simulink model "NL_After_OHC_Function_fil"  (R2019b)
settings: Solver=VariableStepAuto  StartTime=0.0  StopTime=testtime  RelTol=1e-3
InitFcn:
  | NL_After_OHC_Test_Parameters
StopFcn:
  | Verify_NL_After_OHC_Function_fil
undefined symbols (not defined in the file or in its folder): Fs, minR, ohcasym, taumax, taumin
libraries: dspsrcs4 x2, simulink x1, hdlmdlgenlib x1, fillib x1
settings Model: Creator=mblun  LastModifiedBy=t96f346
settings OptimizationCC: BlockReduction=off  ConditionallyExecuteInputs=off  DefaultParameterBehavior=Inlined
settings DebuggingCC: AlgebraicLoopMsg=error  InheritedTsInSrcMsg=none
settings HardwareCC: ProdBitPerPointer=32  ProdBitPerSizeT=32  ProdBitPerPtrDiffT=32  ProdLargestAtomicFloat=None  ProdIntDivRoundTo=Undefined  ProdEndianess=Unspecified  ProdWordSize=32  ProdHWDeviceType=ASIC/FPGA->ASIC/FPGA  TargetBitPerPointer=64  TargetBitPerSizeT=64  TargetBitPerPtrDiffT=64  TargetLongLongMode=on  TargetIntDivRoundTo=Zero  TargetEndianess=LittleEndian  TargetWordSize=64  TargetHWDeviceType=Custom Processor->MATLAB Host Computer  ProdEqTarget=off
settings SFSimCC: CustomCodeUndefinedFunction=UseInterfaceOnly

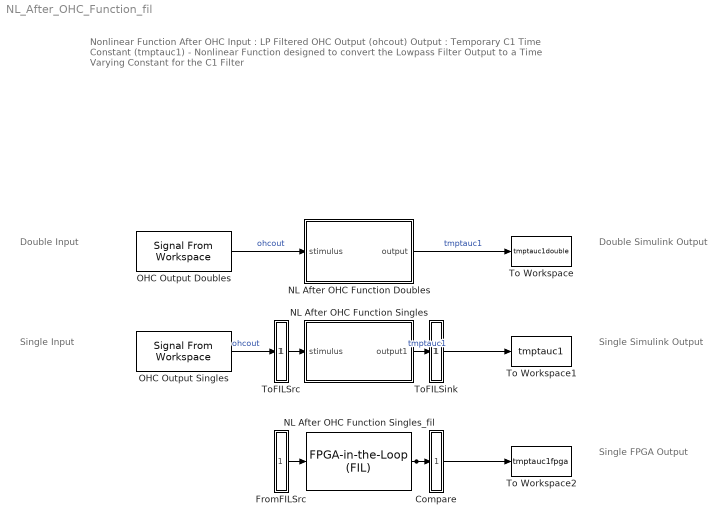
== system NL_After_OHC_Function_fil ==
  note: Nonlinear Function After OHC
      |
      | Input : LP Filtered OHC Output (ohcout)
      |
      | Output : Temporary C1 Time Constant (tmptauc1)
      |
      | - Nonlinear Function designed to convert the Lowpass Filter Output to a Time Varying Constant for the C1 Filter
  note: Single Input
  note: Double Input
  note: Single Simulink Output
  note: Double Simulink Output
  note: Single FPGA Output
  Compare : Subsystem
      mask Display: disp('')
  FromFILSrc : Subsystem
      mask Display: disp('')
  NL After OHC Function Doubles : Subsystem
  NL After OHC Function Singles : Subsystem
  NL After OHC Function Singles_fil : fillib/FPGA-in-the-Loop (FIL)  ForceInterfaceUpdate=0.91338
      settings: SourceProductName=HDL Coder  SourceProductBaseCode=HD
  OHC Output Doubles : dspsrcs4/Signal From Workspace  X=RxSignalDouble  Ts=1/Fs  nsamps=1  OutputAfterFinalValue=Setting to zero  ignoreOrWarnInputAndFrameLengths=off  OutputFrames=off
  OHC Output Singles : dspsrcs4/Signal From Workspace  X=RxSignal  Ts=1/Fs  nsamps=1  OutputAfterFinalValue=Setting to zero  ignoreOrWarnInputAndFrameLengths=off  OutputFrames=off
  To Workspace : ToWorkspace  VariableName=tmptauc1double  SampleTime=-1
      settings: Save2DSignal=2-D array (concatenate along first dimension)
  To Workspace1 : ToWorkspace  VariableName=tmptauc1  SampleTime=-1
      settings: Save2DSignal=2-D array (concatenate along first dimension)
  To Workspace2 : ToWorkspace  VariableName=tmptauc1fpga  SampleTime=-1
      settings: Save2DSignal=2-D array (concatenate along first dimension)
  ToFILSink : Subsystem
      mask Display: disp('')
  ToFILSrc : Subsystem
      mask Display: disp('')
  wires:
  OHC Output Doubles/1 -> NL After OHC Function Doubles/1(stimulus)  "ohcout"
  NL After OHC Function Doubles/1(output) -> To Workspace/1  "tmptauc1"
  ToFILSrc/1(out1) -> NL After OHC Function Singles/1(stimulus)
  NL After OHC Function Singles/1(output1) -> ToFILSink/1(in1)  "tmptauc1"
  OHC Output Singles/1 -> ToFILSrc/1(in1)  "ohcout"
  ToFILSink/1(out1) -> To Workspace1/1
  FromFILSrc/1(out1) -> NL After OHC Function Singles_fil/1
  NL After OHC Function Singles_fil/1 -> To Workspace2/1, Compare/1(in1)

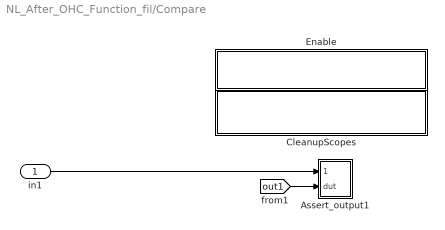
== system NL_After_OHC_Function_fil/Compare ==
  in1 : Inport
  Assert_output1 : Subsystem  mask{ToleranceValue=1e-07}
  CleanupScopes : Subsystem
      settings: OpenFcn=|
      | blkName = gcb; %self block
      | idx = regexp(blkName, '/CleanupScopes$', 'once');
      | blkParent = blkName(1:idx-1);
      | blks=find_system(blkParent, 'LookUnderMasks', 'all','blocktype', 'Scope');
      | for itr = 1:length(blks)
      | 	 hScopeCfg = get_param(blks{itr},'ScopeConfiguration');
      | 	 hScopeCfg.Visible = ~ hScopeCfg.Visible;
      | end
      | drawnow;
      mask Display: fprintf(message('hdlcoder:cosim:vnl_dblclick').getString());
  Enable : Subsystem
      settings: OpenFcn=|
      | blkName = gcb;
      | idx = regexp(blkName, '/Enable$', 'once');
      | blkParent = blkName(1:idx-1);
      | blks=find_system(blkParent, 'LookUnderMasks', 'all','blocktype', 'Assertion');
      | e = get_param(blks{1}, 'Enabled');
      | if strcmp(e, 'on'), f= 'off';, else, f = 'on';, end
      | for ii=1:length(blks), set_param(blks{ii}, 'Enabled', f);, end
      | set_param(gcb, 'MaskDisplay',['fprintf(message(''hdlcoder:cosim:vnl_dblclick_assertions'',','''',upper(e),'''',').getString())']);
      mask Display: fprintf(message('hdlcoder:cosim:vnl_dblclick_assertions','OFF').getString());
  wires:
  in1/1 -> Assert_output1/1(cosim)
  [out1] -> Assert_output1/2(dut)

== system NL_After_OHC_Function_fil/FromFILSrc ==
  dtc1 : DataTypeConversion  OutDataTypeStr=single  SaturateOnIntegerOverflow=on  RndMeth=Zero
  out1 : Outport
  wires:
  [in1] -> dtc1/1
  dtc1/1 -> out1/1

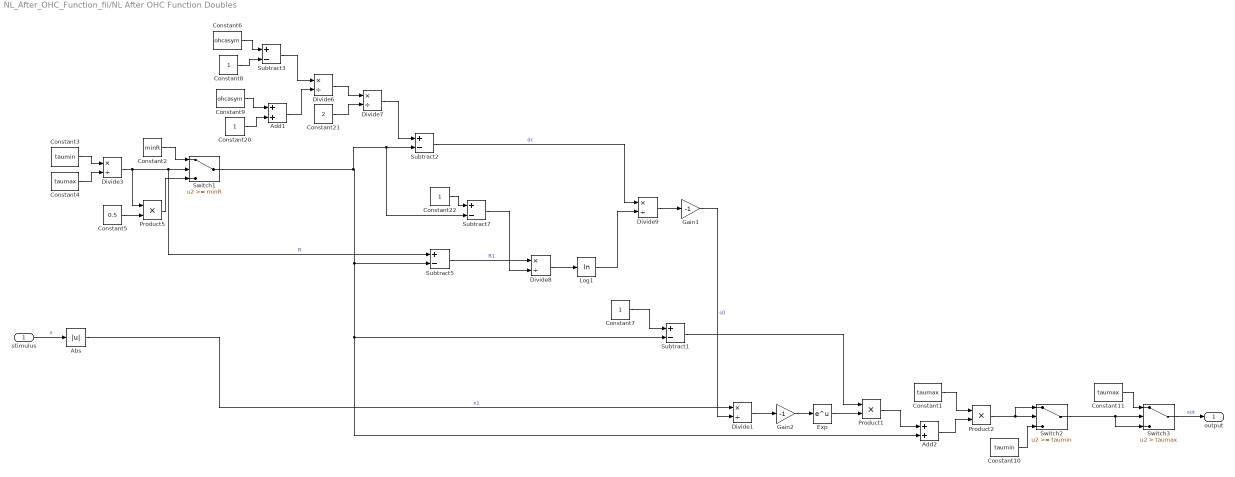
== system NL_After_OHC_Function_fil/NL After OHC Function Doubles ==
  stimulus : Inport
  Abs : Abs
  Add1 : Sum
  Add2 : Sum
  Constant1 : Constant  Value=taumax  SampleTime=-1
  Constant10 : Constant  Value=taumin  SampleTime=-1
  Constant11 : Constant  Value=taumax  SampleTime=-1
  Constant2 : Constant  Value=minR  SampleTime=-1
  Constant{7..8,20,22} (4 alike) : Constant  SampleTime=-1
  Constant21 : Constant  Value=2  SampleTime=-1
  Constant3 : Constant  Value=taumin  SampleTime=-1
  Constant4 : Constant  Value=taumax  SampleTime=-1
  Constant5 : Constant  Value=0.5  SampleTime=-1
  Constant6 : Constant  Value=ohcasym  SampleTime=-1
  Constant9 : Constant  Value=ohcasym  SampleTime=-1
  Divide{1,3,6..9} (6 alike) : Product  Inputs=*/  SaturateOnIntegerOverflow=on  RndMeth=Zero
  Exp : Math  SaturateOnIntegerOverflow=on
  Gain1 : Gain  Gain=-1
  Gain2 : Gain  Gain=-1
  Log1 : Math  Operator=log  SaturateOnIntegerOverflow=on
  Product1 : Product
  Product2 : Product
  Product5 : Product
  Subtract{1..3,5,7} (5 alike) : Sum  Inputs=+-
  Switch1 : Switch  Threshold=minR
  Switch2 : Switch  Threshold=taumin
  Switch3 : Switch  Criteria=u2 > Threshold  Threshold=taumax
  output : Outport  VectorParamsAs1DForOutWhenUnconnected=off
  wires:
  Constant3/1 -> Divide3/1
  Constant4/1 -> Divide3/2
  Divide3/1 -> Subtract5/1, Switch1/2, Product5/1  "R"
  Constant2/1 -> Switch1/1
  Constant5/1 -> Product5/2
  Product5/1 -> Switch1/3
  Switch1/1 -> Subtract7/2, Subtract2/2, Add2/2, Subtract1/2, Subtract5/2
  Constant8/1 -> Subtract3/2
  Constant6/1 -> Subtract3/1
  Constant20/1 -> Add1/2
  Constant9/1 -> Add1/1
  Subtract3/1 -> Divide6/1
  Add1/1 -> Divide6/2
  Divide6/1 -> Divide7/1
  Constant21/1 -> Divide7/2
  Divide7/1 -> Subtract2/1
  Subtract2/1 -> Divide9/1  "dc"
  Subtract5/1 -> Divide8/1  "R1"
  Constant22/1 -> Subtract7/1
  Subtract7/1 -> Divide8/2
  Divide8/1 -> Log1/1
  Log1/1 -> Divide9/2
  Divide9/1 -> Gain1/1
  Gain1/1 -> Divide1/2  "s0"
  stimulus/1 -> Abs/1  "x"
  Abs/1 -> Divide1/1  "x1"
  Constant7/1 -> Subtract1/1
  Divide1/1 -> Gain2/1
  Gain2/1 -> Exp/1
  Subtract1/1 -> Product1/1
  Exp/1 -> Product1/2
  Product1/1 -> Add2/1
  Constant1/1 -> Product2/1
  Add2/1 -> Product2/2
  Product2/1 -> Switch2/1, Switch2/2
  Constant10/1 -> Switch2/3
  Switch2/1 -> Switch3/3, Switch3/2
  Constant11/1 -> Switch3/1
  Switch3/1 -> output/1  "out"

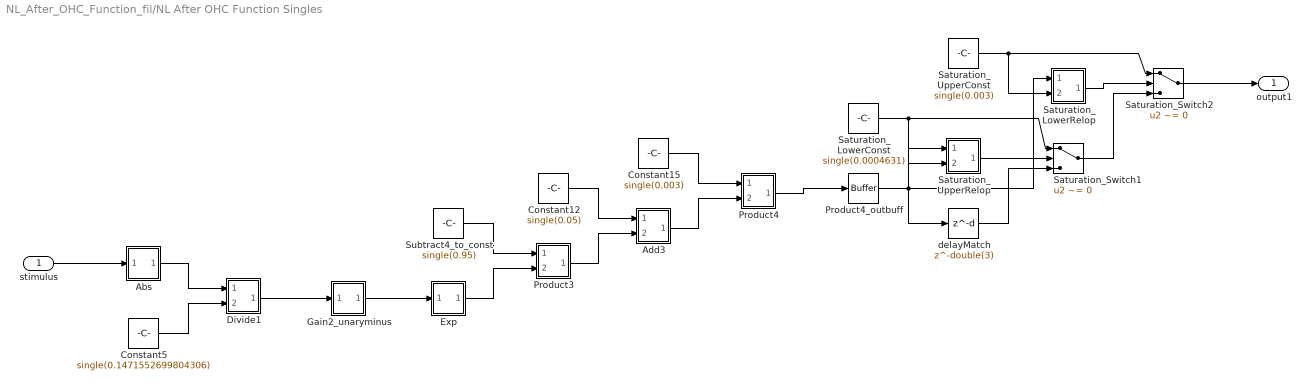
== system NL_After_OHC_Function_fil/NL After OHC Function Singles ==
  stimulus : Inport  OutDataTypeStr=single  PortDimensions=1  SampleTime=2.08333333333333e-05
  Abs : Subsystem
      mask Display: disp('NFP\nabs');
  Add3 : Subsystem
      mask Display: disp('NFP\nadd');
  Constant12 : Constant  Value=single(0.05)  OutDataTypeStr=single  SampleTime=-1
  Constant15 : Constant  Value=single(0.003)  OutDataTypeStr=single  SampleTime=-1
  Constant5 : Constant  Value=single(0.1471552699804306)  OutDataTypeStr=single  SampleTime=-1
  Divide1 : Subsystem
      mask Display: disp('NFP\nmul');
  Exp : Subsystem
      mask Display: disp('NFP\nmath');
  Gain2_unaryminus : Subsystem
      mask Display: disp('NFP\numinus');
  Product3 : Subsystem
      mask Display: disp('NFP\nmul');
  Product4 : Subsystem
      mask Display: disp('NFP\nmul');
  Product4_outbuff : hdlmdlgenlib/Buffer
      settings: SourceProductName=Simulink  SourceProductBaseCode=SL
  Saturation_LowerConst : Constant  Value=single(0.0004631)  OutDataTypeStr=single  SampleTime=-1
  Saturation_LowerRelop : Subsystem
      mask Display: disp('NFP\nrelop');
  Saturation_Switch1 : Switch  Criteria=u2 ~= 0  Threshold=double(0)  OutDataTypeStr=single  SampleTime=2.08333333333333e-05
  Saturation_Switch2 : Switch  Criteria=u2 ~= 0  Threshold=double(0)  OutDataTypeStr=single  SampleTime=2.08333333333333e-05
  Saturation_UpperConst : Constant  Value=single(0.003)  OutDataTypeStr=single  SampleTime=-1
  Saturation_UpperRelop : Subsystem
      mask Display: disp('NFP\nrelop');
  Subtract4_to_const : Constant  Value=single(0.95)  OutDataTypeStr=single  SampleTime=-1
  delayMatch : Delay  DelayLength=double(3)  InitialCondition=0  SampleTime=2.08333333333333e-05
  output1 : Outport  VectorParamsAs1DForOutWhenUnconnected=off
  wires:
  Product4_outbuff/1 -> Saturation_UpperRelop/1(In1), Saturation_LowerRelop/1(In1), delayMatch/1
  Saturation_LowerRelop/1(Out1) -> Saturation_Switch2/2
  Saturation_UpperRelop/1(Out1) -> Saturation_Switch1/2
  Product4/1(Out1) -> Product4_outbuff/1
  Product3/1(Out1) -> Add3/2(In2)
  Exp/1(Out1) -> Product3/2(In2)
  Divide1/1(Out1) -> Gain2_unaryminus/1(In1)
  Add3/1(Out1) -> Product4/2(In2)
  Abs/1(Out1) -> Divide1/1(In1)
  Gain2_unaryminus/1(Out1) -> Exp/1(In1)
  Saturation_Switch1/1 -> Saturation_Switch2/3
  Saturation_UpperConst/1 -> Saturation_Switch2/1, Saturation_LowerRelop/2(In2)
  Saturation_LowerConst/1 -> Saturation_Switch1/1, Saturation_UpperRelop/2(In2)
  Subtract4_to_const/1 -> Product3/1(In1)
  Saturation_Switch2/1 -> output1/1
  delayMatch/1 -> Saturation_Switch1/3
  Constant5/1 -> Divide1/2(In2)
  Constant15/1 -> Product4/1(In1)
  Constant12/1 -> Add3/1(In1)
  stimulus/1 -> Abs/1(In1)

== system NL_After_OHC_Function_fil/ToFILSink ==
  in1 : Inport
  out1 : Outport
  tag scope: out1=global
  wires:
  in1/1 -> out1/1, [out1]

== system NL_After_OHC_Function_fil/ToFILSrc ==
  in1 : Inport
  out1 : Outport
  tag scope: in1=global
  wires:
  in1/1 -> out1/1, [in1]

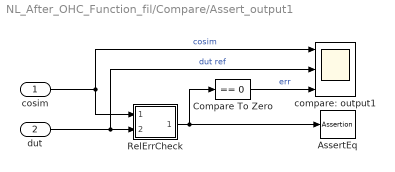
== system NL_After_OHC_Function_fil/Compare/Assert_output1 ==
  cosim : Inport
  dut : Inport  Port=2
  AssertEq : Assertion  StopWhenAssertionFail=off
  Compare To Zero : simulink/Logic and Bit Operations/Compare To Zero  relop===  OutDataTypeStr=boolean
  RelErrCheck : Subsystem
  compare: output1 : Scope  NumInputPorts=3
  wires:
  dut/1 -> compare: output1/2, RelErrCheck/2(In2)  "dut ref"
  cosim/1 -> compare: output1/1, RelErrCheck/1(In1)  "cosim"
  RelErrCheck/1(Out1) -> AssertEq/1, Compare To Zero/1
  Compare To Zero/1 -> compare: output1/3  "err"

== system NL_After_OHC_Function_fil/Compare/CleanupScopes ==

== system NL_After_OHC_Function_fil/Compare/Enable ==

== system NL_After_OHC_Function_fil/NL After OHC Function Singles/Abs ==
  In1 : Inport
  Abs : Abs  SampleTime=2.08333333333333e-05  OutDataTypeStr=single
  Out1 : Outport
  wires:
  Abs/1 -> Out1/1
  In1/1 -> Abs/1

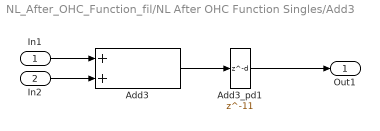
== system NL_After_OHC_Function_fil/NL After OHC Function Singles/Add3 ==
  In1 : Inport
  In2 : Inport  Port=2
  Add3 : Sum  OutDataTypeStr=single  SampleTime=2.08333333333333e-05  SaturateOnIntegerOverflow=on  InputSameDT=on
  Add3_pd1 : Delay  DelayLength=11
  Out1 : Outport
  wires:
  Add3_pd1/1 -> Out1/1
  Add3/1 -> Add3_pd1/1
  In2/1 -> Add3/2
  In1/1 -> Add3/1

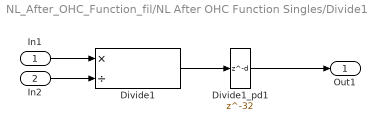
== system NL_After_OHC_Function_fil/NL After OHC Function Singles/Divide1 ==
  In1 : Inport
  In2 : Inport  Port=2
  Divide1 : Product  Inputs=*/  OutDataTypeStr=single  SampleTime=2.08333333333333e-05  SaturateOnIntegerOverflow=on  RndMeth=Zero
  Divide1_pd1 : Delay  DelayLength=32
  Out1 : Outport
  wires:
  Divide1_pd1/1 -> Out1/1
  Divide1/1 -> Divide1_pd1/1
  In2/1 -> Divide1/2
  In1/1 -> Divide1/1

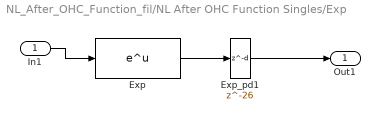
== system NL_After_OHC_Function_fil/NL After OHC Function Singles/Exp ==
  In1 : Inport
  Exp : Math  SampleTime=2.08333333333333e-05  SaturateOnIntegerOverflow=on
  Exp_pd1 : Delay  DelayLength=26
  Out1 : Outport
  wires:
  Exp_pd1/1 -> Out1/1
  Exp/1 -> Exp_pd1/1
  In1/1 -> Exp/1

== system NL_After_OHC_Function_fil/NL After OHC Function Singles/Gain2_unaryminus ==
  In1 : Inport
  Gain2_unaryminus : UnaryMinus  SampleTime=2.08333333333333e-05
  Out1 : Outport
  wires:
  Gain2_unaryminus/1 -> Out1/1
  In1/1 -> Gain2_unaryminus/1

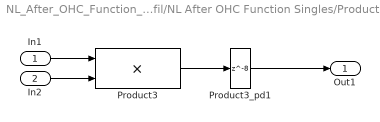
== system NL_After_OHC_Function_fil/NL After OHC Function Singles/Product3 ==
  In1 : Inport
  In2 : Inport  Port=2
  Product3 : Product  Inputs=**  OutDataTypeStr=single  SampleTime=2.08333333333333e-05
  Product3_pd1 : Delay  DelayLength=8
  Out1 : Outport
  wires:
  Product3_pd1/1 -> Out1/1
  Product3/1 -> Product3_pd1/1
  In2/1 -> Product3/2
  In1/1 -> Product3/1

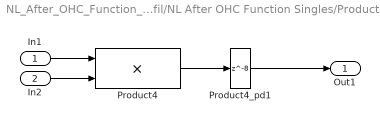
== system NL_After_OHC_Function_fil/NL After OHC Function Singles/Product4 ==
  In1 : Inport
  In2 : Inport  Port=2
  Product4 : Product  Inputs=**  OutDataTypeStr=single  SampleTime=2.08333333333333e-05
  Product4_pd1 : Delay  DelayLength=8
  Out1 : Outport
  wires:
  Product4_pd1/1 -> Out1/1
  Product4/1 -> Product4_pd1/1
  In2/1 -> Product4/2
  In1/1 -> Product4/1

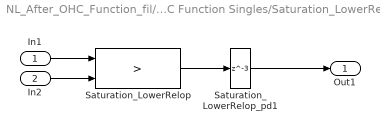
== system NL_After_OHC_Function_fil/NL After OHC Function Singles/Saturation_LowerRelop ==
  In1 : Inport
  In2 : Inport  Port=2
  Saturation_LowerRelop : RelationalOperator  Operator=>  OutDataTypeStr=boolean  SampleTime=2.08333333333333e-05  RndMeth=Nearest
  Saturation_LowerRelop_pd1 : Delay  DelayLength=3
  Out1 : Outport
  wires:
  Saturation_LowerRelop_pd1/1 -> Out1/1
  Saturation_LowerRelop/1 -> Saturation_LowerRelop_pd1/1
  In2/1 -> Saturation_LowerRelop/2
  In1/1 -> Saturation_LowerRelop/1

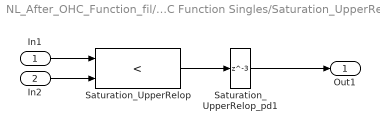
== system NL_After_OHC_Function_fil/NL After OHC Function Singles/Saturation_UpperRelop ==
  In1 : Inport
  In2 : Inport  Port=2
  Saturation_UpperRelop : RelationalOperator  Operator=<  OutDataTypeStr=boolean  SampleTime=2.08333333333333e-05  RndMeth=Nearest
  Saturation_UpperRelop_pd1 : Delay  DelayLength=3
  Out1 : Outport
  wires:
  Saturation_UpperRelop_pd1/1 -> Out1/1
  Saturation_UpperRelop/1 -> Saturation_UpperRelop_pd1/1
  In2/1 -> Saturation_UpperRelop/2
  In1/1 -> Saturation_UpperRelop/1

== system NL_After_OHC_Function_fil/Compare/Assert_output1/RelErrCheck ==
  In1 : Inport
  In2 : Inport  Port=2
  "RelativeErrorCheck " : MATLAB Function  TreatAsAtomicUnit=on
  Out1 : Outport  VectorParamsAs1DForOutWhenUnconnected=off
  wires:
  In2/1 -> "RelativeErrorCheck "/2(R)
  In1/1 -> "RelativeErrorCheck "/1(P)
  "RelativeErrorCheck "/1(y) -> Out1/1

== matlab function NL_After_OHC_Function_fil/Compare/Assert_output1/RelErrCheck/RelativeErrorCheck  ==
  data: P input; y output; R input; ToleranceValue parameter double
% Check if the relative error of R with respect to P is below
% ToleranceValue
% P, R are floating-point
function y = relErrCheck(P,R, ToleranceValue)
    tol = ToleranceValue;
    sz = numel(P);
    assert(sz == numel(R), 'Inputs P and R have different sizes.');
    y = false(1, sz);

    for ii=1:sz
        if (isnan(P(ii)) || isnan(R(ii)))
            if (isnan(P(ii)) && isnan(R(ii)))
                y(ii) = true;
            end
        elseif (isinf(P(ii)) || isinf(R(ii)))
            y(ii) = (P(ii) == R(ii));
        elseif (P(ii) == 0)
            y(ii) = (R(ii) == 0);
        else
            absdiff = abs(P(ii) - R(ii));
            relerr = absdiff/abs(P(ii));
            y(ii) = (relerr <= tol);
        end
    end
end
